simulink library "sm_rollerV_lib_terrain_contact_r5"  (R2026a)
settings: Solver=VariableStepAuto
undefined symbols (not defined in the file): B_Road, CV_Road, F_dyn_Road, F_stat_Road, K_Road, P1, P2, P3, P4, P5, Scene, TW_Road, X, Y, Z
libraries: $bdroot x18, sm_lib x9, sm_trackV_lib_terrain_contact_elem x5, sm_excv_scene_lib x3
Description:
  | Copyright 2024-2026 The MathWorks, Inc.
settings Model: Creator=smiller  LastModifiedBy=smiller

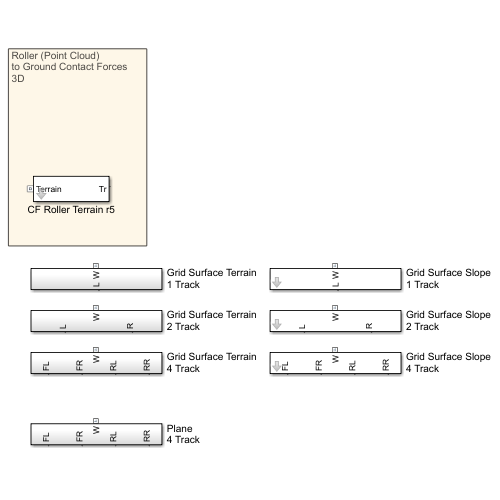
[thumbnail: Simulink's stored preview of the top-level diagram]
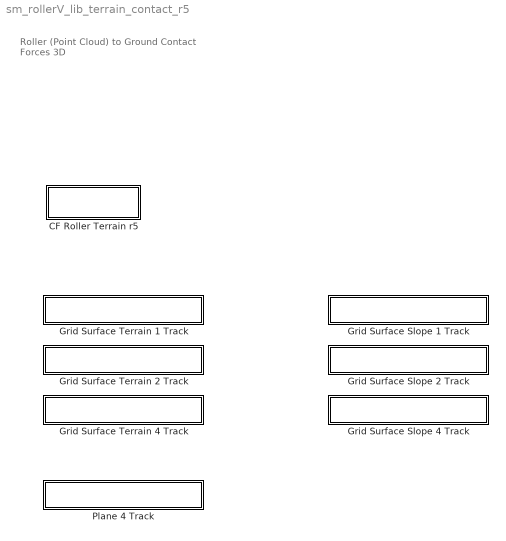
== system sm_rollerV_lib_terrain_contact_r5 ==
  note: Roller (Point Cloud)
      | to Ground Contact Forces
      | 3D
  CF Roller Terrain r5 : Subsystem  mask(Contact Forces, Rollers to Terrain){K_Road=Scene.Contact.Terrain.K, B_Road=Scene.Contact.Terrain.B, TW_Road=Scene.Contact.Terrain.TW, F_dyn_Road=Scene.Contact.Terrain.mud, F_stat_Road=Scene.Contact.Terrain.mus, CV_Road=Scene.Contact.Terrain.CV}
      mask prompts: K_Road "Normal Stiffness (N/m)"; B_Road "Normal Damping (N/(m/s))"; TW_Road "Normal Transition Width (m)"; F_dyn_Road "Coefficient of Dynamic Friction"; F_stat_Road "Coefficient of Static Friction"; CV_Road "Critical Velocity (m/s)"
      mask help: Models contact force between rolling elements and terrain.
  Grid Surface Slope 1 Track : Subsystem  mask{road_len=Scene.Slope.road_len, road_wid=Scene.Slope.road_wid, slope_rise=Scene.Slope.slope_rise, slope_run=Scene.Slope.slope_run, slope_x0=Scene.Slope.slope_start, slope_xres=Scene.Slope.slope_xres, surface_clr=Scene.Slope.clr, surface_opc=Scene.Slope.opc, K_Road=Scene.Contact.Terrain.K, B_Road=Scene.Contact.Terrain.B, TW_Road=Scene.Contact.Terrain.TW, F_dyn_Road=Scene.Contact.Terrain.mud, F_stat_Road=Scene.Contact.Terrain.mus, CV_Road=Scene.Contact.Terrain.CV}
      mask prompts: road_len "Road Length (m)"; road_wid "Road Width (m)"; slope_rise "Slope Rise (m)"; slope_run "Slope Run(m)"; slope_x0 "Slope Start (m)"; slope_xres "Slope Resolution (m)"; surface_clr "Color [R G B] (0-1)"; surface_opc "Opacity (0-1)"; K_Road "Normal Stiffness (N/m)"; B_Road "Normal Damping (N/(m/s))"; TW_Road "Normal Transition Width (m)"; F_dyn_Road "Coefficient of Dynamic Friction"; F_stat_Road "Coefficient of Static Friction"; CV_Road "Critical Velocity (m/s)"
      mask TypeOptions road_len:
      | Grid Surface
      | Slope/road_len
      mask TypeOptions road_wid:
      | Grid Surface
      | Slope/road_wid
      mask TypeOptions slope_rise:
      | Grid Surface
      | Slope/slope_rise
      mask TypeOptions slope_run:
      | Grid Surface
      | Slope/slope_run
      mask TypeOptions slope_x0:
      | Grid Surface
      | Slope/slope_x0
      mask TypeOptions slope_xres:
      | Grid Surface
      | Slope/slope_xres
      mask TypeOptions surface_clr:
      | Grid Surface
      | Slope/surface_clr
      mask TypeOptions surface_opc:
      | Grid Surface
      | Slope/surface_opc
      mask TypeOptions K_Road: CF Track Terrain L/K_Road
      mask TypeOptions B_Road: CF Track Terrain L/B_Road
      mask TypeOptions TW_Road: CF Track Terrain L/TW_Road
      mask TypeOptions F_dyn_Road: CF Track Terrain L/F_dyn_Road
      mask TypeOptions F_stat_Road: CF Track Terrain L/F_stat_Road
      mask TypeOptions CV_Road: CF Track Terrain L/CV_Road
      mask DialogControl cont_slope Prompt: Slope
      mask DialogControl cont_contact Prompt: Contact
  Grid Surface Slope 2 Track : Subsystem  mask{road_len=Scene.Slope.road_len, road_wid=Scene.Slope.road_wid, slope_rise=Scene.Slope.slope_rise, slope_run=Scene.Slope.slope_run, slope_x0=Scene.Slope.slope_start, slope_xres=Scene.Slope.slope_xres, surface_clr=Scene.Slope.clr, surface_opc=Scene.Slope.opc, K_Road=K_Road, B_Road=B_Road, TW_Road=TW_Road, F_dyn_Road=F_dyn_Road, F_stat_Road=F_stat_Road, CV_Road=CV_Road}
      mask prompts: road_len "Road Length (m)"; road_wid "Road Width (m)"; slope_rise "Slope Rise (m)"; slope_run "Slope Run(m)"; slope_x0 "Slope Start (m)"; slope_xres "Slope Resolution (m)"; surface_clr "Color [R G B] (0-1)"; surface_opc "Opacity (0-1)"; K_Road "Normal Stiffness (N/m)"; B_Road "Normal Damping (N/(m/s))"; TW_Road "Normal Transition Width (m)"; F_dyn_Road "Coefficient of Dynamic Friction"; F_stat_Road "Coefficient of Static Friction"; CV_Road "Critical Velocity (m/s)"
      mask TypeOptions road_len:
      | Grid Surface
      | Slope/road_len
      mask TypeOptions road_wid:
      | Grid Surface
      | Slope/road_wid
      mask TypeOptions slope_rise:
      | Grid Surface
      | Slope/slope_rise
      mask TypeOptions slope_run:
      | Grid Surface
      | Slope/slope_run
      mask TypeOptions slope_x0:
      | Grid Surface
      | Slope/slope_x0
      mask TypeOptions slope_xres:
      | Grid Surface
      | Slope/slope_xres
      mask TypeOptions surface_clr:
      | Grid Surface
      | Slope/surface_clr
      mask TypeOptions surface_opc:
      | Grid Surface
      | Slope/surface_opc
      mask TypeOptions K_Road: CF Track Terrain L/K_Road | CF Track Terrain R/K_Road
      mask TypeOptions B_Road: CF Track Terrain L/B_Road | CF Track Terrain R/B_Road
      mask TypeOptions TW_Road: CF Track Terrain L/TW_Road | CF Track Terrain R/TW_Road
      mask TypeOptions F_dyn_Road: CF Track Terrain L/F_dyn_Road | CF Track Terrain R/F_dyn_Road
      mask TypeOptions F_stat_Road: CF Track Terrain L/F_stat_Road | CF Track Terrain R/F_stat_Road
      mask TypeOptions CV_Road: CF Track Terrain L/CV_Road | CF Track Terrain R/CV_Road
      mask DialogControl cont_slope Prompt: Slope
      mask DialogControl cont_contact Prompt: Contact
  Grid Surface Slope 4 Track : Subsystem  mask{road_len=Scene.Slope.road_len, road_wid=Scene.Slope.road_wid, slope_rise=Scene.Slope.slope_rise, slope_run=Scene.Slope.slope_run, slope_x0=Scene.Slope.slope_start, slope_xres=Scene.Slope.slope_xres, surface_clr=Scene.Slope.clr, surface_opc=Scene.Slope.opc, K_Road=Scene.Contact.Terrain.K, B_Road=Scene.Contact.Terrain.B, TW_Road=Scene.Contact.Terrain.TW, F_dyn_Road=Scene.Contact.Terrain.mud, F_stat_Road=Scene.Contact.Terrain.mus, CV_Road=Scene.Contact.Terrain.CV}
      mask prompts: road_len "Road Length (m)"; road_wid "Road Width (m)"; slope_rise "Slope Rise (m)"; slope_run "Slope Run(m)"; slope_x0 "Slope Start (m)"; slope_xres "Slope Resolution (m)"; surface_clr "Color [R G B] (0-1)"; surface_opc "Opacity (0-1)"; K_Road "Normal Stiffness (N/m)"; B_Road "Normal Damping (N/(m/s))"; TW_Road "Normal Transition Width (m)"; F_dyn_Road "Coefficient of Dynamic Friction"; F_stat_Road "Coefficient of Static Friction"; CV_Road "Critical Velocity (m/s)"
      mask TypeOptions road_len:
      | Grid Surface
      | Slope/road_len
      mask TypeOptions road_wid:
      | Grid Surface
      | Slope/road_wid
      mask TypeOptions slope_rise:
      | Grid Surface
      | Slope/slope_rise
      mask TypeOptions slope_run:
      | Grid Surface
      | Slope/slope_run
      mask TypeOptions slope_x0:
      | Grid Surface
      | Slope/slope_x0
      mask TypeOptions slope_xres:
      | Grid Surface
      | Slope/slope_xres
      mask TypeOptions surface_clr:
      | Grid Surface
      | Slope/surface_clr
      mask TypeOptions surface_opc:
      | Grid Surface
      | Slope/surface_opc
      mask TypeOptions K_Road: CF Track Terrain FL/K_Road | CF Track Terrain FR/K_Road | CF Track Terrain RL/K_Road | CF Track Terrain RR/K_Road
      mask TypeOptions B_Road: CF Track Terrain FL/B_Road | CF Track Terrain FR/B_Road | CF Track Terrain RL/B_Road | CF Track Terrain RR/B_Road
      mask TypeOptions TW_Road: CF Track Terrain FL/TW_Road | CF Track Terrain FR/TW_Road | CF Track Terrain RL/TW_Road | CF Track Terrain RR/TW_Road
      mask TypeOptions F_dyn_Road: CF Track Terrain FL/F_dyn_Road | CF Track Terrain FR/F_dyn_Road | CF Track Terrain RL/F_dyn_Road | CF Track Terrain RR/F_dyn_Road
      mask TypeOptions F_stat_Road: CF Track Terrain FL/F_stat_Road | CF Track Terrain FR/F_stat_Road | CF Track Terrain RL/F_stat_Road | CF Track Terrain RR/F_stat_Road
      mask TypeOptions CV_Road: CF Track Terrain FL/CV_Road | CF Track Terrain FR/CV_Road | CF Track Terrain RL/CV_Road | CF Track Terrain RR/CV_Road
      mask DialogControl cont_slope Prompt: Slope
      mask DialogControl cont_contact Prompt: Contact
  Grid Surface Terrain 1 Track : Subsystem
  Grid Surface Terrain 2 Track : Subsystem
  Grid Surface Terrain 4 Track : Subsystem
  Plane 4 Track : Subsystem

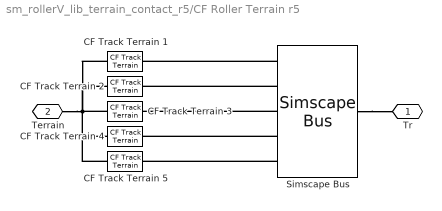
== system sm_rollerV_lib_terrain_contact_r5/CF Roller Terrain r5 ==
  CF Track Terrain {1..5} (5 alike) : sm_trackV_lib_terrain_contact_elem/CF Track Terrain  NormalStiffness=K_Road  NormalDamping=B_Road  NormalTransitionRegionWidth=TW_Road  CoefficientOfDynamicFriction=F_dyn_Road  CoefficientOfStaticFriction=F_stat_Road  FrictionalCriticalVelocity=CV_Road
      settings: LibrarySourceBlock=sm_chain_drive_lib/CF_Road
  Simscape Bus : SimscapeBus  HierarchyStrings=P1;P2;P3;P4;P5  ConnectionType=Bus: CBO_Roller5
  Tr : PMIOPort  Side=Right
  Terrain : PMIOPort  Port=2  Side=Left
  connections:
  CF Track Terrain 1/LConn1 -- CF Track Terrain 2/LConn1 -- CF Track Terrain 5/LConn1 -- CF Track Terrain 4/LConn1 -- Terrain/RConn1 -- CF Track Terrain 3/LConn1
  Simscape Bus/LConn3 -- CF Track Terrain 3/RConn1
  Simscape Bus/LConn2 -- CF Track Terrain 2/RConn1
  Simscape Bus/LConn1 -- CF Track Terrain 1/RConn1
  Simscape Bus/LConn5 -- CF Track Terrain 5/RConn1
  Simscape Bus/LConn4 -- CF Track Terrain 4/RConn1
  Simscape Bus/RConn1 -- Tr/RConn1

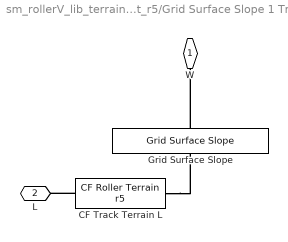
== system sm_rollerV_lib_terrain_contact_r5/Grid Surface Slope 1 Track ==
  CF Track Terrain L : $bdroot/CF Roller Terrain r5  K_Road=K_Road  B_Road=B_Road  TW_Road=TW_Road  F_dyn_Road=F_dyn_Road  F_stat_Road=F_stat_Road  CV_Road=CV_Road
  Grid Surface Slope : sm_excv_scene_lib/Grid Surface Slope  road_len=road_len  road_wid=road_wid  slope_run=slope_run  slope_rise=slope_rise  slope_x0=slope_x0  slope_xres=slope_xres  surface_clr=surface_clr  surface_opc=surface_opc
  W : PMIOPort  Side=Right
  L : PMIOPort  Port=2  Side=Left
  connections:
  CF Track Terrain L/LConn1 -- Grid Surface Slope/LConn1
  Grid Surface Slope/RConn1 -- W/RConn1
  CF Track Terrain L/RConn1 -- L/RConn1

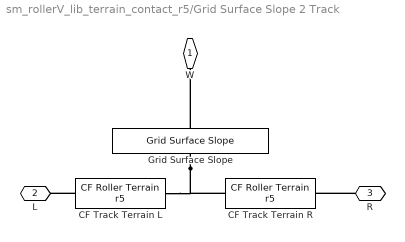
== system sm_rollerV_lib_terrain_contact_r5/Grid Surface Slope 2 Track ==
  CF Track Terrain L : $bdroot/CF Roller Terrain r5  K_Road=K_Road  B_Road=B_Road  TW_Road=TW_Road  F_dyn_Road=F_dyn_Road  F_stat_Road=F_stat_Road  CV_Road=CV_Road
  CF Track Terrain R : $bdroot/CF Roller Terrain r5  K_Road=K_Road  B_Road=B_Road  TW_Road=TW_Road  F_dyn_Road=F_dyn_Road  F_stat_Road=F_stat_Road  CV_Road=CV_Road
  Grid Surface Slope : sm_excv_scene_lib/Grid Surface Slope  road_len=road_len  road_wid=road_wid  slope_run=slope_run  slope_rise=slope_rise  slope_x0=slope_x0  slope_xres=slope_xres  surface_clr=surface_clr  surface_opc=surface_opc
  W : PMIOPort  Side=Right
  L : PMIOPort  Port=2  Side=Left
  R : PMIOPort  Port=3  Side=Left
  connections:
  R/RConn1 -- CF Track Terrain R/RConn1
  CF Track Terrain L/RConn1 -- L/RConn1
  Grid Surface Slope/RConn1 -- W/RConn1
  Grid Surface Slope/LConn1 -- CF Track Terrain R/LConn1 -- CF Track Terrain L/LConn1

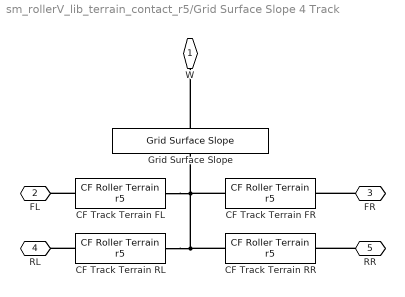
== system sm_rollerV_lib_terrain_contact_r5/Grid Surface Slope 4 Track ==
  CF Track Terrain FL : $bdroot/CF Roller Terrain r5  K_Road=K_Road  B_Road=B_Road  TW_Road=TW_Road  F_dyn_Road=F_dyn_Road  F_stat_Road=F_stat_Road  CV_Road=CV_Road
  CF Track Terrain FR : $bdroot/CF Roller Terrain r5  K_Road=K_Road  B_Road=B_Road  TW_Road=TW_Road  F_dyn_Road=F_dyn_Road  F_stat_Road=F_stat_Road  CV_Road=CV_Road
  CF Track Terrain RL : $bdroot/CF Roller Terrain r5  K_Road=K_Road  B_Road=B_Road  TW_Road=TW_Road  F_dyn_Road=F_dyn_Road  F_stat_Road=F_stat_Road  CV_Road=CV_Road
  CF Track Terrain RR : $bdroot/CF Roller Terrain r5  K_Road=K_Road  B_Road=B_Road  TW_Road=TW_Road  F_dyn_Road=F_dyn_Road  F_stat_Road=F_stat_Road  CV_Road=CV_Road
  Grid Surface Slope : sm_excv_scene_lib/Grid Surface Slope  road_len=road_len  road_wid=road_wid  slope_run=slope_run  slope_rise=slope_rise  slope_x0=slope_x0  slope_xres=slope_xres  surface_clr=surface_clr  surface_opc=surface_opc
  W : PMIOPort  Side=Right
  FL : PMIOPort  Port=2  Side=Left
  FR : PMIOPort  Port=3  Side=Left
  RL : PMIOPort  Port=4  Side=Left
  RR : PMIOPort  Port=5  Side=Left
  connections:
  RR/RConn1 -- CF Track Terrain RR/RConn1
  CF Track Terrain RL/RConn1 -- RL/RConn1
  CF Track Terrain RL/LConn1 -- CF Track Terrain FL/LConn1 -- CF Track Terrain FR/LConn1 -- Grid Surface Slope/LConn1 -- CF Track Terrain RR/LConn1
  Grid Surface Slope/RConn1 -- W/RConn1
  CF Track Terrain FL/RConn1 -- FL/RConn1
  FR/RConn1 -- CF Track Terrain FR/RConn1

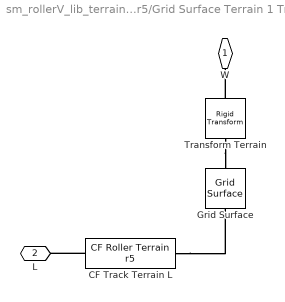
== system sm_rollerV_lib_terrain_contact_r5/Grid Surface Terrain 1 Track ==
  CF Track Terrain L : $bdroot/CF Roller Terrain r5  K_Road=Scene.Contact.Terrain.K  B_Road=Scene.Contact.Terrain.B  TW_Road=Scene.Contact.Terrain.TW  F_dyn_Road=Scene.Contact.Terrain.mud  F_stat_Road=Scene.Contact.Terrain.mus  CV_Road=Scene.Contact.Terrain.CV
  Grid Surface : sm_lib/Curves and Surfaces/Grid Surface  XGridVector=Scene.Terrain.xg  XGridVectorUnits=m  YGridVector=Scene.Terrain.yg  YGridVectorUnits=m  ZHeights=Scene.Terrain.z_heights_data  ZHeightsUnits=m  GraphicType=FromGeometry  GraphicVisPropType=SimpleVisualProperties  GraphicDiffuseColor=[0.8196 0.7255 0.5098]  GraphicOpacity=1.0  GraphicSpecularColor=[0.5 0.5 0.5 1.0]  GraphicAmbientColor=[0.15 0.15 0.15 1.0]  GraphicEmissiveColor=[0.0 0.0 0.0 1.0]  GraphicShininess=75
  Transform Terrain : sm_lib/Frames and Transforms/Rigid Transform  RotationMethod=None  FollAlignAxisA=+X  BaseAlignAxisA=+Y  FollAlignAxisB=+Y  BaseAlignAxisB=+Z  RotationStandardAxis=+Z  RotationAngle=0.0  RotationAngleUnits=deg  RotationArbitraryAxis=[0 0 1]  RotationSequenceAxes=FollowerAxes  RotationSequence=XYX  RotationSequenceAngles=[0 0 0]  RotationSequenceAnglesUnits=deg  RotationMatrix=[1 0 0; 0 1 0; 0 0 1]  Quaternion=[1 0 0 0]  TranslationMethod=Cartesian  TranslationCartesianOffset="[-45 -45+2.5  -2.75+0.2]"  TranslationCartesianOffsetUnits=m  TranslationStandardAxis=+Z  TranslationStandardOffset=0  TranslationStandardOffsetUnits=m  TranslationROffset=0  TranslationROffsetUnits=m  TranslationThetaOffset=0  TranslationThetaOffsetUnits=deg  TranslationZOffset=0  TranslationZOffsetUnits=m
  W : PMIOPort  Side=Right
  L : PMIOPort  Port=2  Side=Left
  connections:
  Transform Terrain/RConn1 -- Grid Surface/LConn1
  CF Track Terrain L/LConn1 -- Grid Surface/RConn1
  Transform Terrain/LConn1 -- W/RConn1
  CF Track Terrain L/RConn1 -- L/RConn1

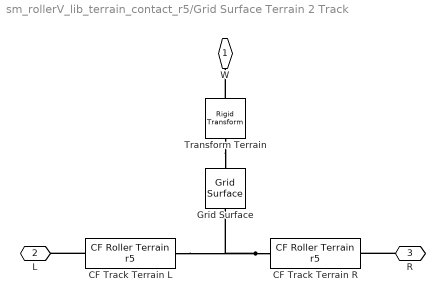
== system sm_rollerV_lib_terrain_contact_r5/Grid Surface Terrain 2 Track ==
  CF Track Terrain L : $bdroot/CF Roller Terrain r5  K_Road=Scene.Contact.Terrain.K  B_Road=Scene.Contact.Terrain.B  TW_Road=Scene.Contact.Terrain.TW  F_dyn_Road=Scene.Contact.Terrain.mud  F_stat_Road=Scene.Contact.Terrain.mus  CV_Road=Scene.Contact.Terrain.CV
  CF Track Terrain R : $bdroot/CF Roller Terrain r5  K_Road=Scene.Contact.Terrain.K  B_Road=Scene.Contact.Terrain.B  TW_Road=Scene.Contact.Terrain.TW  F_dyn_Road=Scene.Contact.Terrain.mud  F_stat_Road=Scene.Contact.Terrain.mus  CV_Road=Scene.Contact.Terrain.CV
  Grid Surface : sm_lib/Curves and Surfaces/Grid Surface  XGridVector=Scene.Terrain.xg  XGridVectorUnits=m  YGridVector=Scene.Terrain.yg  YGridVectorUnits=m  ZHeights=Scene.Terrain.z_heights_data  ZHeightsUnits=m  GraphicType=FromGeometry  GraphicVisPropType=SimpleVisualProperties  GraphicDiffuseColor=[0.8196 0.7255 0.5098]  GraphicOpacity=1.0  GraphicSpecularColor=[0.5 0.5 0.5 1.0]  GraphicAmbientColor=[0.15 0.15 0.15 1.0]  GraphicEmissiveColor=[0.0 0.0 0.0 1.0]  GraphicShininess=75
  Transform Terrain : sm_lib/Frames and Transforms/Rigid Transform  RotationMethod=None  FollAlignAxisA=+X  BaseAlignAxisA=+Y  FollAlignAxisB=+Y  BaseAlignAxisB=+Z  RotationStandardAxis=+Z  RotationAngle=0.0  RotationAngleUnits=deg  RotationArbitraryAxis=[0 0 1]  RotationSequenceAxes=FollowerAxes  RotationSequence=XYX  RotationSequenceAngles=[0 0 0]  RotationSequenceAnglesUnits=deg  RotationMatrix=[1 0 0; 0 1 0; 0 0 1]  Quaternion=[1 0 0 0]  TranslationMethod=Cartesian  TranslationCartesianOffset="[-45 -45+2.5  -2.75+0.2]"  TranslationCartesianOffsetUnits=m  TranslationStandardAxis=+Z  TranslationStandardOffset=0  TranslationStandardOffsetUnits=m  TranslationROffset=0  TranslationROffsetUnits=m  TranslationThetaOffset=0  TranslationThetaOffsetUnits=deg  TranslationZOffset=0  TranslationZOffsetUnits=m
  W : PMIOPort  Side=Right
  L : PMIOPort  Port=2  Side=Left
  R : PMIOPort  Port=3  Side=Left
  connections:
  R/RConn1 -- CF Track Terrain R/RConn1
  CF Track Terrain L/RConn1 -- L/RConn1
  Transform Terrain/LConn1 -- W/RConn1
  CF Track Terrain R/LConn1 -- Grid Surface/RConn1 -- CF Track Terrain L/LConn1
  Transform Terrain/RConn1 -- Grid Surface/LConn1

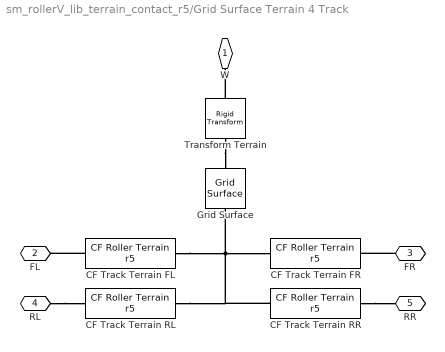
== system sm_rollerV_lib_terrain_contact_r5/Grid Surface Terrain 4 Track ==
  CF Track Terrain FL : $bdroot/CF Roller Terrain r5  K_Road=Scene.Contact.Terrain.K  B_Road=Scene.Contact.Terrain.B  TW_Road=Scene.Contact.Terrain.TW  F_dyn_Road=Scene.Contact.Terrain.mud  F_stat_Road=Scene.Contact.Terrain.mus  CV_Road=Scene.Contact.Terrain.CV
  CF Track Terrain FR : $bdroot/CF Roller Terrain r5  K_Road=Scene.Contact.Terrain.K  B_Road=Scene.Contact.Terrain.B  TW_Road=Scene.Contact.Terrain.TW  F_dyn_Road=Scene.Contact.Terrain.mud  F_stat_Road=Scene.Contact.Terrain.mus  CV_Road=Scene.Contact.Terrain.CV
  CF Track Terrain RL : $bdroot/CF Roller Terrain r5  K_Road=Scene.Contact.Terrain.K  B_Road=Scene.Contact.Terrain.B  TW_Road=Scene.Contact.Terrain.TW  F_dyn_Road=Scene.Contact.Terrain.mud  F_stat_Road=Scene.Contact.Terrain.mus  CV_Road=Scene.Contact.Terrain.CV
  CF Track Terrain RR : $bdroot/CF Roller Terrain r5  K_Road=Scene.Contact.Terrain.K  B_Road=Scene.Contact.Terrain.B  TW_Road=Scene.Contact.Terrain.TW  F_dyn_Road=Scene.Contact.Terrain.mud  F_stat_Road=Scene.Contact.Terrain.mus  CV_Road=Scene.Contact.Terrain.CV
  Grid Surface : sm_lib/Curves and Surfaces/Grid Surface  XGridVector=Scene.Terrain.xg  XGridVectorUnits=m  YGridVector=Scene.Terrain.yg  YGridVectorUnits=m  ZHeights=Scene.Terrain.z_heights_data  ZHeightsUnits=m  GraphicType=FromGeometry  GraphicVisPropType=SimpleVisualProperties  GraphicDiffuseColor=[0.8196 0.7255 0.5098]  GraphicOpacity=1.0  GraphicSpecularColor=[0.5 0.5 0.5 1.0]  GraphicAmbientColor=[0.15 0.15 0.15 1.0]  GraphicEmissiveColor=[0.0 0.0 0.0 1.0]  GraphicShininess=75
  Transform Terrain : sm_lib/Frames and Transforms/Rigid Transform  RotationMethod=None  FollAlignAxisA=+X  BaseAlignAxisA=+Y  FollAlignAxisB=+Y  BaseAlignAxisB=+Z  RotationStandardAxis=+Z  RotationAngle=0.0  RotationAngleUnits=deg  RotationArbitraryAxis=[0 0 1]  RotationSequenceAxes=FollowerAxes  RotationSequence=XYX  RotationSequenceAngles=[0 0 0]  RotationSequenceAnglesUnits=deg  RotationMatrix=[1 0 0; 0 1 0; 0 0 1]  Quaternion=[1 0 0 0]  TranslationMethod=Cartesian  TranslationCartesianOffset="[-45 -45+2.5  -2.75+0.2]"  TranslationCartesianOffsetUnits=m  TranslationStandardAxis=+Z  TranslationStandardOffset=0  TranslationStandardOffsetUnits=m  TranslationROffset=0  TranslationROffsetUnits=m  TranslationThetaOffset=0  TranslationThetaOffsetUnits=deg  TranslationZOffset=0  TranslationZOffsetUnits=m
  W : PMIOPort  Side=Right
  FL : PMIOPort  Port=2  Side=Left
  FR : PMIOPort  Port=3  Side=Left
  RL : PMIOPort  Port=4  Side=Left
  RR : PMIOPort  Port=5  Side=Left
  connections:
  CF Track Terrain RR/RConn1 -- RR/RConn1
  RL/RConn1 -- CF Track Terrain RL/RConn1
  Transform Terrain/RConn1 -- Grid Surface/LConn1
  CF Track Terrain FL/LConn1 -- Grid Surface/RConn1 -- CF Track Terrain RR/LConn1 -- CF Track Terrain RL/LConn1 -- CF Track Terrain FR/LConn1
  Transform Terrain/LConn1 -- W/RConn1
  CF Track Terrain FL/RConn1 -- FL/RConn1
  FR/RConn1 -- CF Track Terrain FR/RConn1

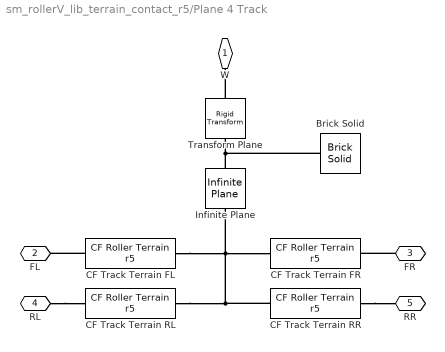
== system sm_rollerV_lib_terrain_contact_r5/Plane 4 Track ==
  Brick Solid : sm_lib/Body Elements/Brick Solid  BrickDimensions=[36 33 0.05]  BrickDimensionsUnits=m  ExportEntireGeometry=off  InertiaType=CalculateFromGeometry  BasedOnType=Density  Density=1000  DensityUnits=kg/m^3  Mass=1  MassUnits=kg  CenterOfMass=[0 0 0]  CenterOfMassUnits=m  MomentsOfInertia=[1 1 1]  MomentsOfInertiaUnits=kg*m^2  ProductsOfInertia=[0 0 0]  ProductsOfInertiaUnits=kg*m^2  GraphicType=FromGeometry  MarkerShape=Sphere  MarkerSize=10  GraphicVisPropType=SimpleVisualProperties  GraphicDiffuseColor=[0.8196 0.7255 0.5098]  GraphicOpacity=1.0  GraphicSpecularColor=[0.5 0.5 0.5 1.0]  GraphicAmbientColor=[0.15 0.15 0.15 1.0]  GraphicEmissiveColor=[0.0 0.0 0.0 1.0]  GraphicShininess=75  DoExposeReferenceFrame=off  SerializedFrames=<Frames><Frame><Id>Frame1</Id><Value><Name>Top</Name><Origin><Source>GeometricFeature</Source><FeatureName>+z surface</FeatureName></Origin><PrimaryAxis><DefinedDirection>+Z</DefinedDirection><Source>ReferenceFrame</Source><SourceDirection>+Z</SourceDirection><FeatureName></FeatureName></PrimaryAxis><SecondaryAxis><DefinedDirection>+X</DefinedDirection><Source>ReferenceFrame</Source><SourceDirection>+X</SourceDirection><FeatureName></FeatureName></SecondaryAxis></Value></Frame></Frames>
  CF Track Terrain FL : $bdroot/CF Roller Terrain r5  K_Road=Scene.Contact.Terrain.K  B_Road=Scene.Contact.Terrain.B  TW_Road=Scene.Contact.Terrain.TW  F_dyn_Road=Scene.Contact.Terrain.mud  F_stat_Road=Scene.Contact.Terrain.mus  CV_Road=Scene.Contact.Terrain.CV
  CF Track Terrain FR : $bdroot/CF Roller Terrain r5  K_Road=Scene.Contact.Terrain.K  B_Road=Scene.Contact.Terrain.B  TW_Road=Scene.Contact.Terrain.TW  F_dyn_Road=Scene.Contact.Terrain.mud  F_stat_Road=Scene.Contact.Terrain.mus  CV_Road=Scene.Contact.Terrain.CV
  CF Track Terrain RL : $bdroot/CF Roller Terrain r5  K_Road=Scene.Contact.Terrain.K  B_Road=Scene.Contact.Terrain.B  TW_Road=Scene.Contact.Terrain.TW  F_dyn_Road=Scene.Contact.Terrain.mud  F_stat_Road=Scene.Contact.Terrain.mus  CV_Road=Scene.Contact.Terrain.CV
  CF Track Terrain RR : $bdroot/CF Roller Terrain r5  K_Road=Scene.Contact.Terrain.K  B_Road=Scene.Contact.Terrain.B  TW_Road=Scene.Contact.Terrain.TW  F_dyn_Road=Scene.Contact.Terrain.mud  F_stat_Road=Scene.Contact.Terrain.mus  CV_Road=Scene.Contact.Terrain.CV
  Infinite Plane : sm_lib/Curves and Surfaces/Infinite Plane  GraphicType=None  GraphicPlaneWidth=28  GraphicPlaneWidthUnits=m  GraphicPlaneHeight=40  GraphicPlaneHeightUnits=m  GraphicVisPropType=SimpleVisualProperties  GraphicDiffuseColor=[0.5 0.5 0.5]  GraphicOpacity=0.25  GraphicSpecularColor=[0.5 0.5 0.5 1.0]  GraphicAmbientColor=[0.15 0.15 0.15 1.0]  GraphicEmissiveColor=[0.0 0.0 0.0 1.0]  GraphicShininess=75
  Transform Plane : sm_lib/Frames and Transforms/Rigid Transform  RotationMethod=None  FollAlignAxisA=+X  BaseAlignAxisA=+Y  FollAlignAxisB=+Y  BaseAlignAxisB=+Z  RotationStandardAxis=+Z  RotationAngle=0.0  RotationAngleUnits=deg  RotationArbitraryAxis=[0 0 1]  RotationSequenceAxes=FollowerAxes  RotationSequence=XYX  RotationSequenceAngles=[0 0 0]  RotationSequenceAnglesUnits=deg  RotationMatrix=[1 0 0; 0 1 0; 0 0 1]  Quaternion=[1 0 0 0]  TranslationMethod=Cartesian  TranslationCartesianOffset=[16 14.5 0]  TranslationCartesianOffsetUnits=m  TranslationStandardAxis=+Z  TranslationStandardOffset=0  TranslationStandardOffsetUnits=m  TranslationROffset=0  TranslationROffsetUnits=m  TranslationThetaOffset=0  TranslationThetaOffsetUnits=deg  TranslationZOffset=0  TranslationZOffsetUnits=m
  W : PMIOPort  Side=Right
  FL : PMIOPort  Port=2  Side=Left
  FR : PMIOPort  Port=3  Side=Left
  RL : PMIOPort  Port=4  Side=Left
  RR : PMIOPort  Port=5  Side=Left
  connections:
  Transform Plane/RConn1 -- Brick Solid/LConn1 -- Infinite Plane/LConn1
  FR/RConn1 -- CF Track Terrain FR/RConn1
  CF Track Terrain FL/RConn1 -- FL/RConn1
  Transform Plane/LConn1 -- W/RConn1
  CF Track Terrain RL/LConn1 -- CF Track Terrain FR/LConn1 -- CF Track Terrain FL/LConn1 -- Infinite Plane/RConn1 -- CF Track Terrain RR/LConn1
  RL/RConn1 -- CF Track Terrain RL/RConn1
  CF Track Terrain RR/RConn1 -- RR/RConn1
